simulink model "RocketSimulation"  (R2019b)
settings: Solver=VariableStepAuto  StartTime=0.0  StopTime=10.0  RelTol=1e-3
InitFcn:
  | SimInit;
values from neighbouring files (symbols this model uses):
  AtmoData = [128.186136479 128.244270677 128.302404875 128.485675494 128.734477787 129.006749738 129.455630863 129.904511988 130.470611984 131.122189026 131.781835085 132.638750532 ... (4000 elements, 1000x4)]    [EarthAtmoData.mat]
undefined symbols (not defined in the file or in its folder): Aero_On, AtmoAlt_planet, Cd, Cl, Constant_Drag_On, Constant_Lift_On, Drag_On, DragData, g0, GM_planet, Lift_On, Omega_planet, PitchOverAlt, PitchOverAngle, PitchSwitch, R_planet, RefSurfArea, SimData
libraries: simulink_extras x6, dspmathops x4, vrlib x2, simulink x1
settings Model: Creator=raulm_000  LastModifiedBy=raulm_000

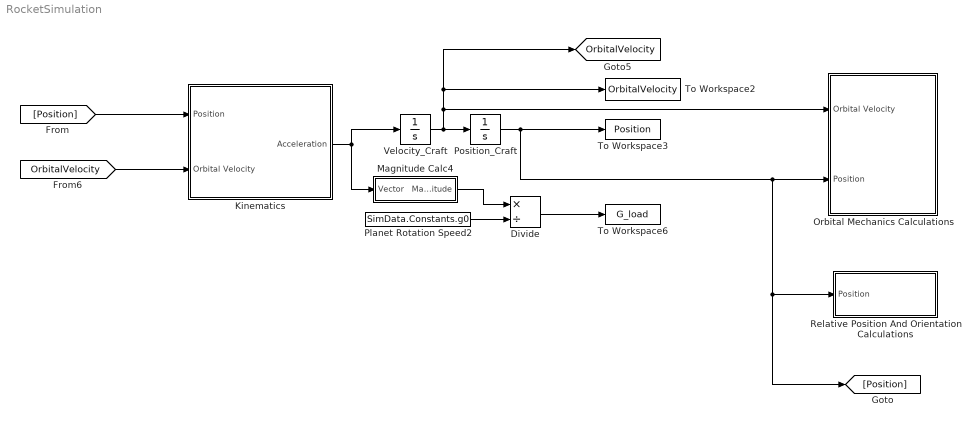
== system RocketSimulation ==
  Divide : Product  Inputs=*/
  Kinematics : Subsystem
  Magnitude Calc4 : Subsystem
  Orbital Mechanics Calculations : Subsystem
  Planet Rotation Speed2 : Constant  Value=SimData.Constants.g0
  Position_Craft : Integrator  InitialCondition=SimData.InitialCondition.P
  Relative Position And Orientation Calculations : Subsystem
  To Workspace2 : ToWorkspace  VariableName=OrbitalVelocity  SampleTime=-1
  To Workspace3 : ToWorkspace  VariableName=Position  SampleTime=-1
  To Workspace6 : ToWorkspace  VariableName=G_load  SampleTime=-1
  Velocity_Craft : Integrator  InitialCondition=SimData.InitialCondition.V
  tag scope: OrbitalVelocity=global
  wires:
  [OrbitalVelocity] -> Kinematics/2(Orbital Velocity)
  Kinematics/1("Acceleration ") -> Velocity_Craft/1, Magnitude Calc4/1(Vector)
  Magnitude Calc4/1("Magnitude ") -> Divide/1
  Planet Rotation Speed2/1 -> Divide/2
  Divide/1 -> To Workspace6/1
  Velocity_Craft/1 -> Position_Craft/1, [OrbitalVelocity], To Workspace2/1, Orbital Mechanics Calculations/1(Orbital Velocity)
  [Position] -> Kinematics/1(Position)
  Position_Craft/1 -> [Position], Relative Position And Orientation Calculations/1(Position), Orbital Mechanics Calculations/2(Position), To Workspace3/1

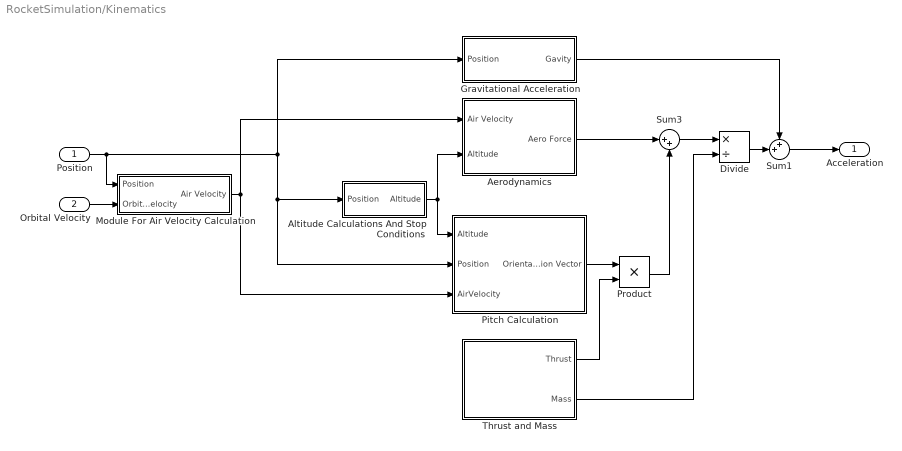
== system RocketSimulation/Kinematics ==
  Position : Inport
  Orbital Velocity : Inport  Port=2
  Aerodynamics : Subsystem
  Altitude Calculations And Stop Conditions : Subsystem
  Divide : Product  Inputs=*/
  Gravitational Acceleration : Subsystem
  Module For Air Velocity Calculation : Subsystem
  Pitch Calculation : Subsystem
  Product : Product
  Sum1 : Sum  Inputs=++|
  Sum3 : Sum  Inputs=|++
  Thrust and Mass : Subsystem
  "Acceleration " : Outport
  wires:
  Position/1 -> Module For Air Velocity Calculation/1(Position), Gravitational Acceleration/1(Position), Pitch Calculation/2(Position), Altitude Calculations And Stop Conditions/1(Position)
  Module For Air Velocity Calculation/1(Air Velocity) -> Pitch Calculation/3(AirVelocity), Aerodynamics/1(Air Velocity)
  Thrust and Mass/1("Thrust ") -> Product/2
  Altitude Calculations And Stop Conditions/1(Altitude) -> Pitch Calculation/1(Altitude), Aerodynamics/2("Altitude ")
  Orbital Velocity/1 -> Module For Air Velocity Calculation/2(Orbital Velocity)
  Pitch Calculation/1(Orientation Vector) -> Product/1
  Aerodynamics/1("Aero Force ") -> Sum3/1
  Product/1 -> Sum3/2
  Sum3/1 -> Divide/1
  Thrust and Mass/2(Mass) -> Divide/2
  Divide/1 -> Sum1/2
  Sum1/1 -> "Acceleration "/1
  Gravitational Acceleration/1("Gavity ") -> Sum1/1

== system RocketSimulation/Magnitude Calc4 ==
  Vector : Inport
  Add : Sum
  Demux : Demux  Outputs=2
  Math Function : Math  Operator=square  SaturateOnIntegerOverflow=on
  Math Function1 : Math  Operator=square  SaturateOnIntegerOverflow=on
  Sqrt : Sqrt  SaturateOnIntegerOverflow=on
  "Magnitude " : Outport
  wires:
  Demux/1 -> Math Function1/1
  Demux/2 -> Math Function/1
  Math Function/1 -> Add/2
  Add/1 -> Sqrt/1
  Vector/1 -> Demux/1
  Math Function1/1 -> Add/1
  Sqrt/1 -> "Magnitude "/1

== system RocketSimulation/Orbital Mechanics Calculations ==
  Orbital Velocity : Inport
  Position : Inport  Port=2
  Gain1 : Gain  Gain=1.01
  MATLAB Function : MATLAB Function  TreatAsAtomicUnit=on
  Planet Rotation Speed4 : Constant  Value=SimData.TargetOrbit
  Relational Operator : RelationalOperator  OutDataTypeStr=boolean  RndMeth=Nearest
  tag scope: TOR=global
  wires:
  Planet Rotation Speed4/1 -> Gain1/1
  Relational Operator/1 -> [TOR]
  Gain1/1 -> Relational Operator/2
  Orbital Velocity/1 -> MATLAB Function/1(OrbitVelocity)
  Position/1 -> MATLAB Function/2(Position)

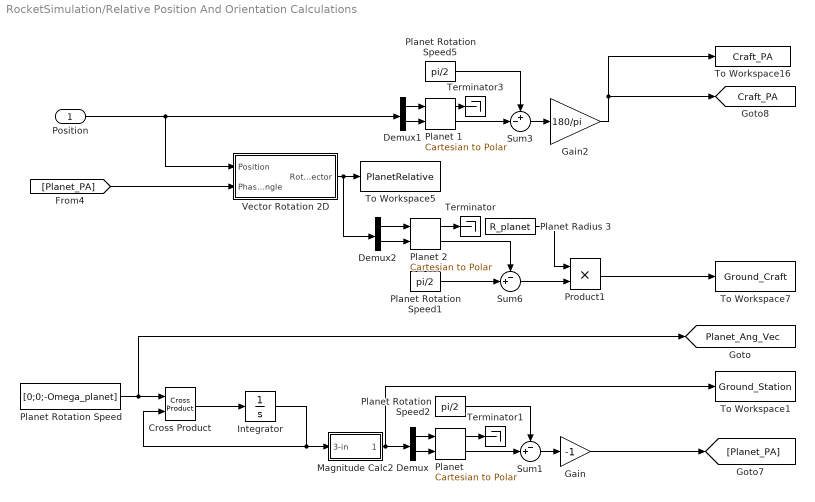
== system RocketSimulation/Relative Position And Orientation Calculations ==
  Position : Inport
  Cross Product : vrlib/Utilities/Cross Product
      settings: SourceProductName=Simulink
  Demux : Demux  Outputs=2
  Demux1 : Demux  Outputs=2
  Demux2 : Demux  Outputs=2
  Gain : Gain  Gain=-1
  Gain2 : Gain  Gain=180/pi
  Integrator : Integrator  InitialCondition=[0;R_planet;0]
  Magnitude Calc2 : Subsystem
  "Planet " : simulink_extras/Transformations/Cartesian to Polar
      settings: SourceProductName=Simulink
  Planet 1 : simulink_extras/Transformations/Cartesian to Polar
      settings: SourceProductName=Simulink
  Planet 2 : simulink_extras/Transformations/Cartesian to Polar
      settings: SourceProductName=Simulink
  Planet Radius 3 : Constant  Value=R_planet
  Planet Rotation Speed : Constant  Value=[0;0;-Omega_planet]
  Planet Rotation Speed1 : Constant  Value=pi/2
  Planet Rotation Speed2 : Constant  Value=pi/2
  Planet Rotation Speed5 : Constant  Value=pi/2
  Product1 : Product
  Sum1 : Sum  Inputs=-+|
  Sum3 : Sum  Inputs=+-|
  Sum6 : Sum  Inputs=-+|
  Terminator : Terminator
  Terminator1 : Terminator
  Terminator3 : Terminator
  To Workspace1 : ToWorkspace  VariableName=Ground_Station  SampleTime=-1
  To Workspace16 : ToWorkspace  VariableName=Craft_PA  SampleTime=-1
  To Workspace5 : ToWorkspace  VariableName=PlanetRelative  SampleTime=-1
  To Workspace7 : ToWorkspace  VariableName=Ground_Craft  SampleTime=-1
  Vector Rotation 2D : Subsystem
  tag scope: Craft_PA=global, Planet_Ang_Vec=global
  wires:
  Planet Rotation Speed/1 -> [Planet_Ang_Vec], Cross Product/1
  Integrator/1 -> Cross Product/2, Magnitude Calc2/1(3-in)
  Cross Product/1 -> Integrator/1
  Magnitude Calc2/1("2-out ") -> To Workspace1/1, Demux/1
  Demux/1 -> "Planet "/1
  Demux/2 -> "Planet "/2
  Vector Rotation 2D/1("Rotated Vector ") -> Demux2/1, To Workspace5/1
  "Planet "/2 -> Sum1/2
  Planet Rotation Speed2/1 -> Sum1/1
  Sum1/1 -> Gain/1
  Planet 2/2 -> Sum6/1
  Planet Radius 3/1 -> Product1/1
  Product1/1 -> To Workspace7/1
  Planet Rotation Speed1/1 -> Sum6/2
  Sum6/1 -> Product1/2
  Demux2/1 -> Planet 2/1
  Demux2/2 -> Planet 2/2
  Planet 2/1 -> Terminator/1
  "Planet "/1 -> Terminator1/1
  Gain/1 -> [Planet_PA]
  [Planet_PA] -> Vector Rotation 2D/2(Phase Angle)
  Demux1/1 -> Planet 1/1
  Demux1/2 -> Planet 1/2
  Planet 1/2 -> Sum3/2
  Planet Rotation Speed5/1 -> Sum3/1
  Planet 1/1 -> Terminator3/1
  Sum3/1 -> Gain2/1
  Gain2/1 -> To Workspace16/1, [Craft_PA]
  Position/1 -> Vector Rotation 2D/1(Position), Demux1/1

== system RocketSimulation/Kinematics/Aerodynamics ==
  Air Velocity : Inport
  "Altitude " : Inport  Port=2
  Add : Sum  Inputs=+-
  Aerodynamic Calculations : Subsystem
  Atmosphere Max Alt : Constant  Value=AtmoAlt_planet
  Constant1 : Constant  Value=0
  Constant2 : Constant  Value=Aero_On
  Constant3 : Constant  Value=0
  Switch : Switch  Criteria=u2 > Threshold
  Switch1 : Switch  Criteria=u2 ~= 0
  "Aero Force " : Outport
  wires:
  "Altitude "/1 -> Aerodynamic Calculations/2(Altitude), Add/2
  Atmosphere Max Alt/1 -> Add/1
  Add/1 -> Switch/2
  Constant1/1 -> Switch/3
  Switch1/1 -> "Aero Force "/1
  Air Velocity/1 -> Aerodynamic Calculations/1(Air Velocity)
  Aerodynamic Calculations/1("Aeroforce ") -> Switch/1
  Switch/1 -> Switch1/3
  Constant2/1 -> Switch1/2
  Constant3/1 -> Switch1/1

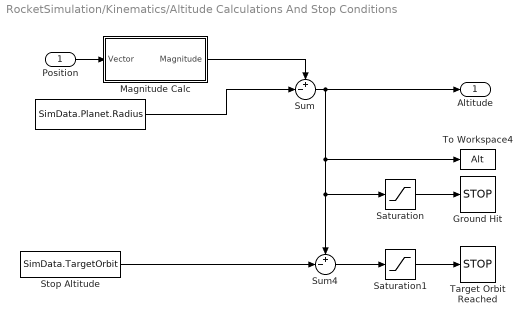
== system RocketSimulation/Kinematics/Altitude Calculations And Stop Conditions ==
  Position : Inport
  " " : Constant  Value=SimData.Planet.Radius
  " Target Orbit Reached" : Stop
  Ground Hit : Stop
  Magnitude Calc : Subsystem
  Saturation : Saturate  UpperLimit=0
  Saturation1 : Saturate  UpperLimit=1  LowerLimit=0
  Stop Altitude : Constant  Value=SimData.TargetOrbit
  Sum : Sum  Inputs=+-|
  Sum4 : Sum  Inputs=+-|
  To Workspace4 : ToWorkspace  VariableName=Alt  SampleTime=-1
  Altitude : Outport
  wires:
  Magnitude Calc/1("Magnitude ") -> Sum/1
  " "/1 -> Sum/2
  Sum/1 -> Sum4/1, Saturation/1, To Workspace4/1, Altitude/1
  Saturation/1 -> Ground Hit/1
  Stop Altitude/1 -> Sum4/2
  Sum4/1 -> Saturation1/1
  Saturation1/1 -> " Target Orbit Reached"/1
  Position/1 -> Magnitude Calc/1(Vector)

== system RocketSimulation/Kinematics/Gravitational Acceleration ==
  Position : Inport
  Divide : Product  Inputs=*/
  Gain : Gain  Gain=-1
  Magnitude Calc : Subsystem
  Math Function : Math  Operator=square  SaturateOnIntegerOverflow=on
  Normalization : dspmathops/Normalization  NormType=2-norm  Bias=1e-10  NormOver=Specified dimension  Dimension=1  roundingMode=Floor  overflowMode=off  accumDataTypeStr=Inherit: Same as product output  accumLastDataTypeStr=Inherit: Same as product output  outputDataTypeStr=Inherit: Same as product output  outputMin=[]  outputMax=[]  outputLastDataTypeStr=Inherit: Same as product output
      settings: SourceProductName=DSP System Toolbox
  Planet GM : Constant  Value=GM_planet
  Product : Product
  "Gavity " : Outport
  wires:
  Position/1 -> Normalization/1, Magnitude Calc/1(Vector)
  Magnitude Calc/1("Magnitude ") -> Math Function/1
  Planet GM/1 -> Divide/1
  Math Function/1 -> Divide/2
  Product/1 -> "Gavity "/1
  Gain/1 -> Product/2
  Divide/1 -> Product/1
  Normalization/1 -> Gain/1

== system RocketSimulation/Kinematics/Module For Air Velocity Calculation ==
  Position : Inport
  Orbital Velocity : Inport  Port=2
  Cross Product1 : vrlib/Utilities/Cross Product
      settings: SourceProductName=Simulink
  Magnitude Calc3 : Subsystem
  Mux : Mux  Inputs=2
  Planet Rotation Speed1 : Constant  Value=0
  Sum2 : Sum  Inputs=|-+
  Air Velocity : Outport
  wires:
  [Planet_Ang_Vec] -> Cross Product1/1
  Cross Product1/1 -> Magnitude Calc3/1(3-in)
  Mux/1 -> Cross Product1/2
  Planet Rotation Speed1/1 -> Mux/2
  Magnitude Calc3/1("2-out ") -> Sum2/1
  Orbital Velocity/1 -> Sum2/2
  Position/1 -> Mux/1
  Sum2/1 -> Air Velocity/1

== system RocketSimulation/Kinematics/Pitch Calculation ==
  Altitude : Inport  PortDimensions=1
  Position : Inport  Port=2
  AirVelocity : Inport  Port=3
  Constant : Constant  Value=PitchOverAlt
  Gravity Turn Pitch Calculation : Subsystem
  Relational Operator : RelationalOperator  OutDataTypeStr=boolean  RndMeth=Nearest
  Subsystem : Subsystem
  Switch1 : Switch  Criteria=u2 ~= 0  Threshold=PitchOverAlt
  Orientation Vector : Outport
  wires:
  Relational Operator/1 -> Switch1/2
  Constant/1 -> Relational Operator/1
  Altitude/1 -> Subsystem/2(Altitude), Relational Operator/2
  Switch1/1 -> Orientation Vector/1
  Position/1 -> Subsystem/1(Position)
  Subsystem/1(Up Vector) -> Switch1/1
  AirVelocity/1 -> Gravity Turn Pitch Calculation/1(Air Velocity)
  Gravity Turn Pitch Calculation/1(Thrust Vec) -> Switch1/3

== system RocketSimulation/Kinematics/Thrust and Mass ==
  Mass and fuel consumption : Subsystem
  To Workspace1 : ToWorkspace  VariableName=Mass  SampleTime=-1
  "Thrust " : Outport
  Mass : Outport  Port=2
  wires:
  Mass and fuel consumption/1("Thrust ") -> "Thrust "/1
  Mass and fuel consumption/2("Mass ") -> To Workspace1/1, Mass/1

== system RocketSimulation/Relative Position And Orientation Calculations/Magnitude Calc2 ==
  3-in : Inport
  Demux4 : Demux  Outputs=3
  Mux2 : Mux  Inputs=2
  Terminator3 : Terminator
  "2-out " : Outport
  wires:
  3-in/1 -> Demux4/1
  Demux4/3 -> Terminator3/1
  Demux4/1 -> Mux2/1
  Demux4/2 -> Mux2/2
  Mux2/1 -> "2-out "/1

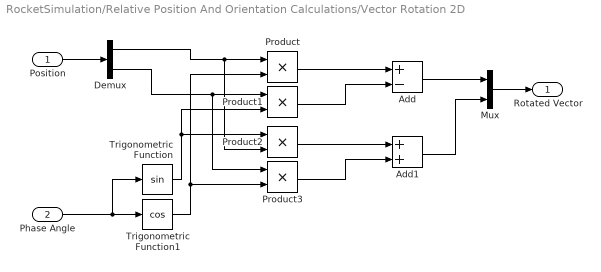
== system RocketSimulation/Relative Position And Orientation Calculations/Vector Rotation 2D ==
  Position : Inport
  Phase Angle : Inport  Port=2
  Add : Sum  Inputs=+-
  Add1 : Sum
  Demux : Demux  Outputs=2
  Mux : Mux  Inputs=2
  Product{,1..3} (4 alike) : Product
  Trigonometric Function : Trigonometry
  Trigonometric Function1 : Trigonometry  Operator=cos
  "Rotated Vector " : Outport
  wires:
  Mux/1 -> "Rotated Vector "/1
  Phase Angle/1 -> Trigonometric Function/1, Trigonometric Function1/1
  Position/1 -> Demux/1
  Trigonometric Function1/1 -> Product3/2, Product/2
  Demux/1 -> Product2/2, Product/1
  Product/1 -> Add/1
  Demux/2 -> Product3/1, Product1/1
  Trigonometric Function/1 -> Product2/1, Product1/2
  Product1/1 -> Add/2
  Product2/1 -> Add1/1
  Product3/1 -> Add1/2
  Add1/1 -> Mux/2
  Add/1 -> Mux/1

== system RocketSimulation/Kinematics/Aerodynamics/Aerodynamic Calculations ==
  Air Velocity : Inport
  Altitude : Inport  Port=2
  Cl and Cd Calculation : Subsystem
  Magnitude Calc1 : Subsystem
  Product : Product  Inputs=3
  Referance Surface Area : Constant  Value=RefSurfArea
  "Aeroforce " : Outport
  wires:
  Air Velocity/1 -> Cl and Cd Calculation/1(Air Velocity), Magnitude Calc1/1(Air Velocity)
  Altitude/1 -> Cl and Cd Calculation/2("Altitude "), Magnitude Calc1/2("Altitude ")
  Product/1 -> "Aeroforce "/1
  Magnitude Calc1/1("Dynamic Pressure ") -> Product/1
  Cl and Cd Calculation/1(Cl + Cd) -> Product/2
  Referance Surface Area/1 -> Product/3

== system RocketSimulation/Kinematics/Altitude Calculations And Stop Conditions/Magnitude Calc ==
  Vector : Inport
  Add : Sum
  Demux : Demux  Outputs=2
  Math Function : Math  Operator=square  SaturateOnIntegerOverflow=on
  Math Function1 : Math  Operator=square  SaturateOnIntegerOverflow=on
  Sqrt : Sqrt  SaturateOnIntegerOverflow=on
  "Magnitude " : Outport
  wires:
  Demux/1 -> Math Function1/1
  Demux/2 -> Math Function/1
  Math Function/1 -> Add/2
  Add/1 -> Sqrt/1
  Vector/1 -> Demux/1
  Math Function1/1 -> Add/1
  Sqrt/1 -> "Magnitude "/1

== system RocketSimulation/Kinematics/Gravitational Acceleration/Magnitude Calc ==
  Vector : Inport
  Add : Sum
  Demux : Demux  Outputs=2
  Math Function : Math  Operator=square  SaturateOnIntegerOverflow=on
  Math Function1 : Math  Operator=square  SaturateOnIntegerOverflow=on
  Sqrt : Sqrt  SaturateOnIntegerOverflow=on
  "Magnitude " : Outport
  wires:
  Demux/1 -> Math Function1/1
  Demux/2 -> Math Function/1
  Math Function/1 -> Add/2
  Add/1 -> Sqrt/1
  Vector/1 -> Demux/1
  Math Function1/1 -> Add/1
  Sqrt/1 -> "Magnitude "/1

== system RocketSimulation/Kinematics/Module For Air Velocity Calculation/Magnitude Calc3 ==
  3-in : Inport
  Demux4 : Demux  Outputs=3
  Mux2 : Mux  Inputs=2
  Terminator3 : Terminator
  "2-out " : Outport
  wires:
  3-in/1 -> Demux4/1
  Demux4/3 -> Terminator3/1
  Demux4/1 -> Mux2/1
  Demux4/2 -> Mux2/2
  Mux2/1 -> "2-out "/1

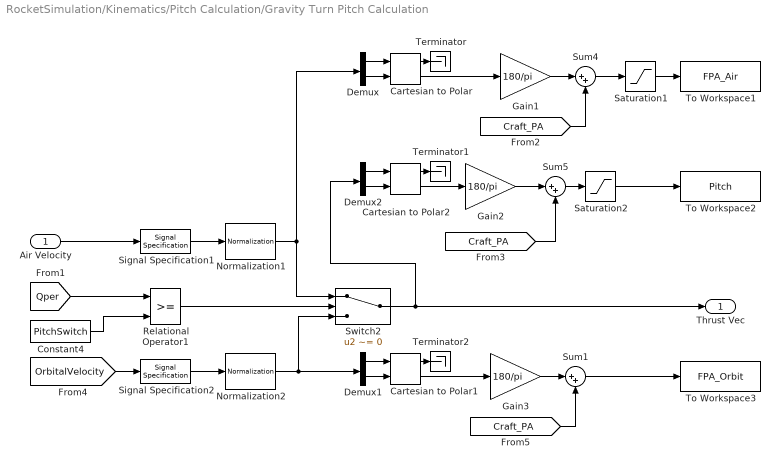
== system RocketSimulation/Kinematics/Pitch Calculation/Gravity Turn Pitch Calculation ==
  Air Velocity : Inport
  Cartesian to Polar : simulink_extras/Transformations/Cartesian to Polar
      settings: SourceProductName=Simulink
  Cartesian to Polar1 : simulink_extras/Transformations/Cartesian to Polar
      settings: SourceProductName=Simulink
  Cartesian to Polar2 : simulink_extras/Transformations/Cartesian to Polar
      settings: SourceProductName=Simulink
  Constant4 : Constant  Value=PitchSwitch
  Demux : Demux  Outputs=2
  Demux1 : Demux  Outputs=2
  Demux2 : Demux  Outputs=2
  Gain1 : Gain  Gain=180/pi
  Gain2 : Gain  Gain=180/pi
  Gain3 : Gain  Gain=180/pi
  Normalization1 : dspmathops/Normalization  NormType=2-norm  Bias=1e-10  NormOver=Specified dimension  Dimension=1  roundingMode=Floor  overflowMode=off  accumDataTypeStr=Inherit: Same as product output  accumLastDataTypeStr=Inherit: Same as product output  outputMin=[]  outputMax=[]
      settings: SourceProductName=DSP System Toolbox
  Normalization2 : dspmathops/Normalization  NormType=2-norm  Bias=1e-10  NormOver=Specified dimension  Dimension=1  roundingMode=Floor  overflowMode=off  accumDataTypeStr=Inherit: Same as product output  accumLastDataTypeStr=Inherit: Same as product output  outputMin=[]  outputMax=[]
      settings: SourceProductName=DSP System Toolbox
  Relational Operator1 : RelationalOperator  OutDataTypeStr=boolean  RndMeth=Nearest
  Saturation1 : Saturate  UpperLimit=90  LowerLimit=0
  Saturation2 : Saturate  UpperLimit=90  LowerLimit=0
  Signal Specification1 : SignalSpecification  Dimensions=2
  Signal Specification2 : SignalSpecification  Dimensions=2
  Sum1 : Sum  Inputs=|++
  Sum4 : Sum  Inputs=|++
  Sum5 : Sum  Inputs=|++
  Switch2 : Switch  Criteria=u2 ~= 0  Threshold=PitchOverAlt
  Terminator : Terminator
  Terminator1 : Terminator
  Terminator2 : Terminator
  To Workspace1 : ToWorkspace  VariableName=FPA_Air  SampleTime=-1
  To Workspace2 : ToWorkspace  VariableName=Pitch  SampleTime=-1
  To Workspace3 : ToWorkspace  VariableName=FPA_Orbit  SampleTime=-1
  Thrust Vec : Outport
  wires:
  [Qper] -> Relational Operator1/1
  Relational Operator1/1 -> Switch2/2
  Normalization1/1 -> Switch2/1, Demux/1
  Demux1/1 -> Cartesian to Polar1/1
  Switch2/1 -> Thrust Vec/1, Demux2/1
  Constant4/1 -> Relational Operator1/2
  Cartesian to Polar/1 -> Terminator/1
  Sum1/1 -> To Workspace3/1
  Air Velocity/1 -> Signal Specification1/1
  Demux/2 -> Cartesian to Polar/2
  Signal Specification2/1 -> Normalization2/1
  Normalization2/1 -> Demux1/1, Switch2/3
  Signal Specification1/1 -> Normalization1/1
  Demux/1 -> Cartesian to Polar/1
  Demux1/2 -> Cartesian to Polar1/2
  Cartesian to Polar1/1 -> Terminator2/1
  [OrbitalVelocity] -> Signal Specification2/1
  Gain1/1 -> Sum4/1
  Cartesian to Polar1/2 -> Gain3/1
  Gain3/1 -> Sum1/1
  [Craft_PA] -> Sum1/2
  Saturation2/1 -> To Workspace2/1
  Cartesian to Polar/2 -> Gain1/1
  Cartesian to Polar2/1 -> Terminator1/1
  Saturation1/1 -> To Workspace1/1
  Gain2/1 -> Sum5/1
  [Craft_PA] -> Sum5/2
  Sum5/1 -> Saturation2/1
  Demux2/1 -> Cartesian to Polar2/1
  Cartesian to Polar2/2 -> Gain2/1
  Demux2/2 -> Cartesian to Polar2/2
  [Craft_PA] -> Sum4/2
  Sum4/1 -> Saturation1/1

== system RocketSimulation/Kinematics/Pitch Calculation/Subsystem ==
  Position : Inport
  Altitude : Inport  Port=2
  Gain : Gain  Gain=-pi/180
  Linear Pitch Over : Gain  Gain=PitchOverAngle/PitchOverAlt
  Normalization : dspmathops/Normalization  NormType=2-norm  Bias=1e-10  NormOver=Specified dimension  Dimension=1  roundingMode=Floor  overflowMode=off  accumDataTypeStr=Inherit: Same as product output  accumLastDataTypeStr=Inherit: Same as product output  outputMin=[]  outputMax=[]
      settings: SourceProductName=DSP System Toolbox
  Saturation : Saturate  UpperLimit=90  LowerLimit=0
  Signal Specification : SignalSpecification  Dimensions=2
  Vector Rotation 2D : Subsystem
  Up Vector : Outport
  wires:
  Altitude/1 -> Linear Pitch Over/1
  Position/1 -> Signal Specification/1
  Signal Specification/1 -> Normalization/1
  Normalization/1 -> Vector Rotation 2D/1(Position)
  Saturation/1 -> Gain/1
  Gain/1 -> Vector Rotation 2D/2(Phase Angle)
  Linear Pitch Over/1 -> Saturation/1
  Vector Rotation 2D/1("Rotated Vector ") -> Up Vector/1

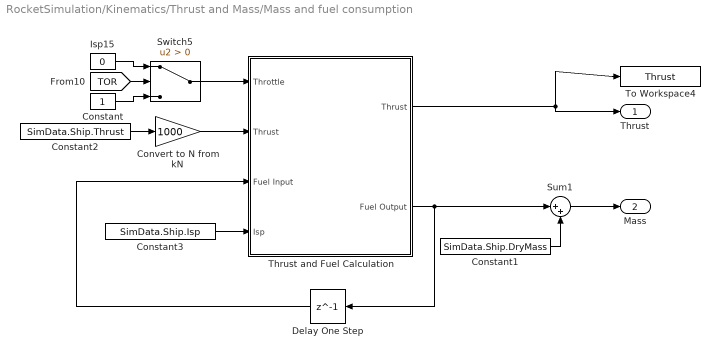
== system RocketSimulation/Kinematics/Thrust and Mass/Mass and fuel consumption ==
  Constant : Constant
  Constant1 : Constant  Value=SimData.Ship.DryMass
  Constant2 : Constant  Value=SimData.Ship.Thrust
  Constant3 : Constant  Value=SimData.Ship.Isp
  Convert to N from kN : Gain  Gain=1000
  Delay One Step : Delay  DelayLength=1
  Isp15 : Constant  Value=0
  Sum1 : Sum  Inputs=|++
  Switch5 : Switch  Criteria=u2 > Threshold
  Thrust and Fuel Calculation : Subsystem
  To Workspace4 : ToWorkspace  VariableName=Thrust  SampleTime=-1
      settings: MaxDataPoints=1
  "Thrust " : Outport
  "Mass " : Outport  Port=2
  wires:
  Sum1/1 -> "Mass "/1
  Convert to N from kN/1 -> Thrust and Fuel Calculation/2(Thrust)
  Thrust and Fuel Calculation/1("Thrust ") -> "Thrust "/1, To Workspace4/1
  Thrust and Fuel Calculation/2(Fuel Output) -> Delay One Step/1, Sum1/1
  Isp15/1 -> Switch5/1
  [TOR] -> Switch5/2
  Constant/1 -> Switch5/3
  Switch5/1 -> Thrust and Fuel Calculation/1(Throttle)
  Delay One Step/1 -> Thrust and Fuel Calculation/3(Fuel Input)
  Constant1/1 -> Sum1/2
  Constant2/1 -> Convert to N from kN/1
  Constant3/1 -> Thrust and Fuel Calculation/4(Isp)

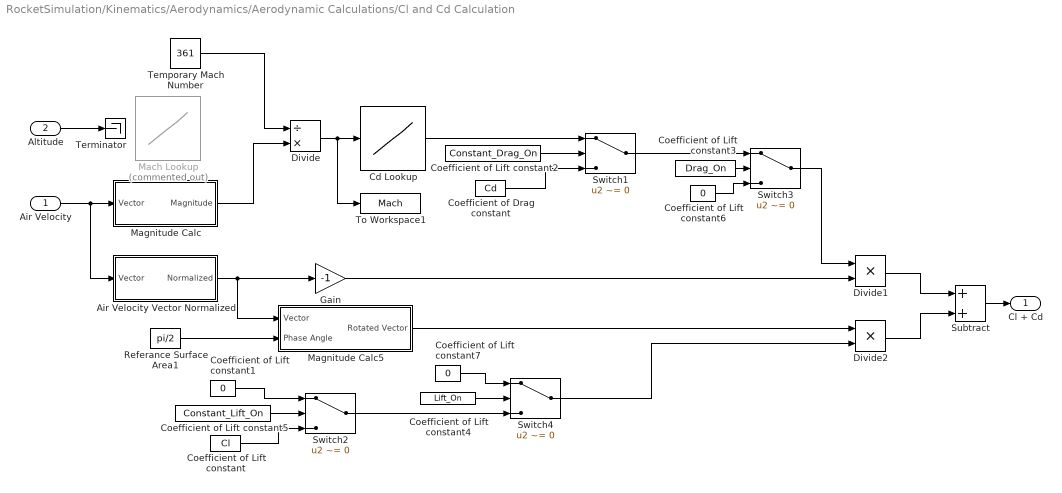
== system RocketSimulation/Kinematics/Aerodynamics/Aerodynamic Calculations/Cl and Cd Calculation ==
  Air Velocity : Inport
  "Altitude " : Inport  Port=2
  Air Velocity Vector Normalized : Subsystem
  Cd Lookup : Lookup_n-D  NumberOfTableDimensions=1  BreakpointsForDimension1=DragData(:,1)  Table=DragData(:,2)  InternalRulePriority=Speed  RndMeth=Simplest  InputSameDT=on
  Coefficient of Drag constant : Constant  Value=Cd
  Coefficient of Lift constant : Constant  Value=Cl
  Coefficient of Lift constant1 : Constant  Value=0
  Coefficient of Lift constant2 : Constant  Value=Constant_Drag_On
  Coefficient of Lift constant3 : Constant  Value=Drag_On
  Coefficient of Lift constant4 : Constant  Value=Lift_On
  Coefficient of Lift constant5 : Constant  Value=Constant_Lift_On
  Coefficient of Lift constant6 : Constant  Value=0
  Coefficient of Lift constant7 : Constant  Value=0
  Divide : Product  Inputs=/*
  Divide1 : Product  Inputs=**
  Divide2 : Product  Inputs=**
  Gain : Gain  Gain=-1
  Mach Lookup : Lookup_n-D  Commented=on  NumberOfTableDimensions=1  BreakpointsForDimension1=AtmoData(:,1)  Table=AtmoData(:,4)  InternalRulePriority=Speed  RndMeth=Simplest  InputSameDT=on
  Magnitude Calc : Subsystem
  Magnitude Calc5 : Subsystem
  Referance Surface Area1 : Constant  Value=pi/2
  Subtract : Sum
  Switch{1..4} (4 alike) : Switch  Criteria=u2 ~= 0
  Temporary Mach Number : Constant  Value=361
  Terminator : Terminator
  To Workspace1 : ToWorkspace  VariableName=Mach  SampleTime=-1
  Cl + Cd : Outport
  wires:
  Air Velocity/1 -> Air Velocity Vector Normalized/1(Vector), Magnitude Calc/1(Vector)
  Magnitude Calc/1("Magnitude ") -> Divide/2
  Divide/1 -> To Workspace1/1, Cd Lookup/1
  Air Velocity Vector Normalized/1("Normalized ") -> Magnitude Calc5/1(Vector), Gain/1
  Gain/1 -> Divide1/2
  Divide1/1 -> Subtract/1
  Referance Surface Area1/1 -> Magnitude Calc5/2(Phase Angle)
  Magnitude Calc5/1("Rotated Vector ") -> Divide2/1
  Coefficient of Lift constant2/1 -> Switch1/2
  Switch3/1 -> Divide1/1
  Subtract/1 -> Cl + Cd/1
  Coefficient of Drag constant/1 -> Switch1/3
  Cd Lookup/1 -> Switch1/1
  Coefficient of Lift constant5/1 -> Switch2/2
  Coefficient of Lift constant1/1 -> Switch2/1
  Coefficient of Lift constant/1 -> Switch2/3
  Coefficient of Lift constant3/1 -> Switch3/2
  Coefficient of Lift constant6/1 -> Switch3/3
  Switch1/1 -> Switch3/1
  Coefficient of Lift constant4/1 -> Switch4/2
  Switch2/1 -> Switch4/3
  Coefficient of Lift constant7/1 -> Switch4/1
  Switch4/1 -> Divide2/2
  Divide2/1 -> Subtract/2
  "Altitude "/1 -> Terminator/1
  Temporary Mach Number/1 -> Divide/1

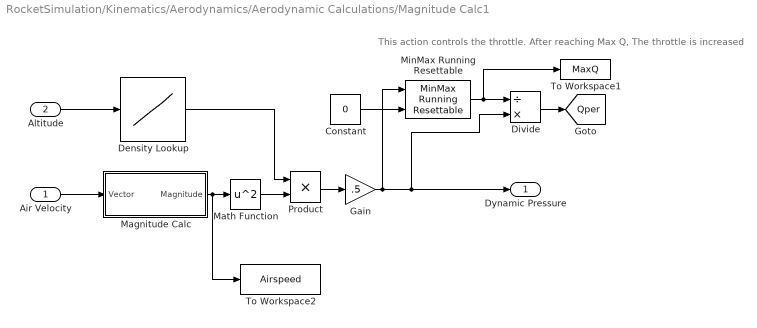
== system RocketSimulation/Kinematics/Aerodynamics/Aerodynamic Calculations/Magnitude Calc1 ==
  note: This action controls the throttle. After reaching Max Q, The throttle is increased
  Air Velocity : Inport
  "Altitude " : Inport  Port=2
  Constant : Constant  Value=0
  Density Lookup : Lookup_n-D  NumberOfTableDimensions=1  BreakpointsForDimension1=AtmoData(:,1)  Table=AtmoData(:,3)  InternalRulePriority=Speed  RndMeth=Simplest  InputSameDT=on
  Divide : Product  Inputs=/*
  Gain : Gain  Gain=.5
  Magnitude Calc : Subsystem
  Math Function : Math  Operator=square  SaturateOnIntegerOverflow=on
  MinMax Running Resettable : simulink/Math Operations/MinMax Running Resettable  Function=max  vinit=0.0
  Product : Product
  To Workspace1 : ToWorkspace  VariableName=MaxQ  SampleTime=-1
      settings: MaxDataPoints=1
  To Workspace2 : ToWorkspace  VariableName=Airspeed  SampleTime=-1
  "Dynamic Pressure " : Outport
  tag scope: Qper=global
  wires:
  "Altitude "/1 -> Density Lookup/1
  Magnitude Calc/1("Magnitude ") -> To Workspace2/1, Math Function/1
  Air Velocity/1 -> Magnitude Calc/1(Vector)
  Math Function/1 -> Product/2
  Product/1 -> Gain/1
  Density Lookup/1 -> Product/1
  MinMax Running Resettable/1 -> To Workspace1/1, Divide/1
  Constant/1 -> MinMax Running Resettable/2
  Gain/1 -> MinMax Running Resettable/1, Divide/2, "Dynamic Pressure "/1
  Divide/1 -> [Qper]

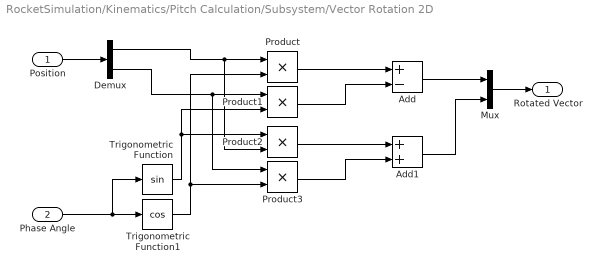
== system RocketSimulation/Kinematics/Pitch Calculation/Subsystem/Vector Rotation 2D ==
  Position : Inport
  Phase Angle : Inport  Port=2
  Add : Sum  Inputs=+-
  Add1 : Sum
  Demux : Demux  Outputs=2
  Mux : Mux  Inputs=2
  Product{,1..3} (4 alike) : Product
  Trigonometric Function : Trigonometry
  Trigonometric Function1 : Trigonometry  Operator=cos
  "Rotated Vector " : Outport
  wires:
  Mux/1 -> "Rotated Vector "/1
  Phase Angle/1 -> Trigonometric Function/1, Trigonometric Function1/1
  Position/1 -> Demux/1
  Trigonometric Function1/1 -> Product3/2, Product/2
  Demux/1 -> Product2/2, Product/1
  Product/1 -> Add/1
  Demux/2 -> Product3/1, Product1/1
  Trigonometric Function/1 -> Product2/1, Product1/2
  Product1/1 -> Add/2
  Product2/1 -> Add1/1
  Product3/1 -> Add1/2
  Add1/1 -> Mux/2
  Add/1 -> Mux/1

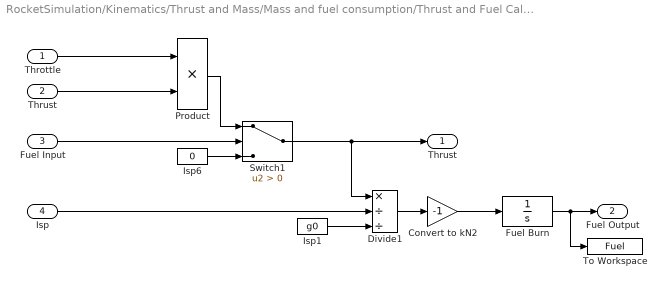
== system RocketSimulation/Kinematics/Thrust and Mass/Mass and fuel consumption/Thrust and Fuel Calculation ==
  Throttle : Inport
  Thrust : Inport  Port=2
  Fuel Input : Inport  Port=3
  Isp : Inport  Port=4
  Convert to kN2 : Gain  Gain=-1
  Divide1 : Product  Inputs=*//
  Fuel Burn : Integrator  InitialCondition=SimData.Ship.WetMass - SimData.Ship.DryMass  LimitOutput=on  LowerSaturationLimit=0
  Isp1 : Constant  Value=g0
  Isp6 : Constant  Value=0
  Product : Product
  Switch1 : Switch  Criteria=u2 > Threshold
  To Workspace : ToWorkspace  VariableName=Fuel  SampleTime=-1
      settings: MaxDataPoints=1
  "Thrust " : Outport
  Fuel Output : Outport  Port=2
  wires:
  Isp1/1 -> Divide1/3
  Divide1/1 -> Convert to kN2/1
  Convert to kN2/1 -> Fuel Burn/1
  Thrust/1 -> Product/2
  Product/1 -> Switch1/1
  Throttle/1 -> Product/1
  Switch1/1 -> Divide1/1, "Thrust "/1
  Isp6/1 -> Switch1/3
  Isp/1 -> Divide1/2
  Fuel Input/1 -> Switch1/2
  Fuel Burn/1 -> Fuel Output/1, To Workspace/1

== system RocketSimulation/Kinematics/Aerodynamics/Aerodynamic Calculations/Cl and Cd Calculation/Air Velocity Vector Normalized ==
  Vector : Inport
  Constant : Constant
  Demux3 : Demux  Outputs=2
  Divide1 : Product  Inputs=*/
  Divide2 : Product  Inputs=*/
  Magnitude Calc : Subsystem
  Mux1 : Mux  Inputs=2
  Switch : Switch  Criteria=u2 > Threshold
  "Normalized " : Outport
  wires:
  Demux3/1 -> Divide1/1
  Vector/1 -> Demux3/1, Magnitude Calc/1(Vector)
  Mux1/1 -> "Normalized "/1
  Demux3/2 -> Divide2/1
  Constant/1 -> Switch/3
  Magnitude Calc/1("Magnitude ") -> Switch/1
  Magnitude Calc/2(Is Zero) -> Switch/2
  Divide1/1 -> Mux1/1
  Divide2/1 -> Mux1/2
  Switch/1 -> Divide2/2, Divide1/2

== system RocketSimulation/Kinematics/Aerodynamics/Aerodynamic Calculations/Cl and Cd Calculation/Magnitude Calc ==
  Vector : Inport
  Add : Sum
  Demux : Demux  Outputs=2
  Math Function : Math  Operator=square  SaturateOnIntegerOverflow=on
  Math Function1 : Math  Operator=square  SaturateOnIntegerOverflow=on
  Sqrt : Sqrt  SaturateOnIntegerOverflow=on
  "Magnitude " : Outport
  wires:
  Demux/1 -> Math Function1/1
  Demux/2 -> Math Function/1
  Math Function/1 -> Add/2
  Add/1 -> Sqrt/1
  Vector/1 -> Demux/1
  Math Function1/1 -> Add/1
  Sqrt/1 -> "Magnitude "/1

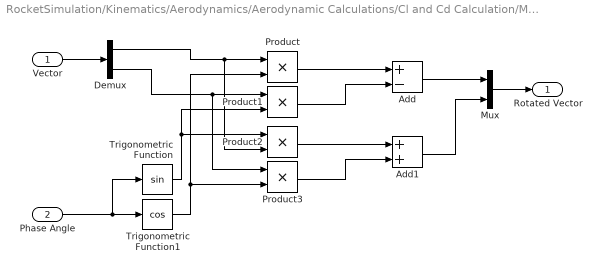
== system RocketSimulation/Kinematics/Aerodynamics/Aerodynamic Calculations/Cl and Cd Calculation/Magnitude Calc5 ==
  Vector : Inport
  Phase Angle : Inport  Port=2
  Add : Sum  Inputs=+-
  Add1 : Sum
  Demux : Demux  Outputs=2
  Mux : Mux  Inputs=2
  Product{,1..3} (4 alike) : Product
  Trigonometric Function : Trigonometry
  Trigonometric Function1 : Trigonometry  Operator=cos
  "Rotated Vector " : Outport
  wires:
  Mux/1 -> "Rotated Vector "/1
  Phase Angle/1 -> Trigonometric Function/1, Trigonometric Function1/1
  Vector/1 -> Demux/1
  Trigonometric Function1/1 -> Product3/2, Product/2
  Demux/1 -> Product2/2, Product/1
  Product/1 -> Add/1
  Demux/2 -> Product3/1, Product1/1
  Trigonometric Function/1 -> Product2/1, Product1/2
  Product1/1 -> Add/2
  Product2/1 -> Add1/1
  Product3/1 -> Add1/2
  Add1/1 -> Mux/2
  Add/1 -> Mux/1

== system RocketSimulation/Kinematics/Aerodynamics/Aerodynamic Calculations/Magnitude Calc1/Magnitude Calc ==
  Vector : Inport
  Add : Sum
  Demux : Demux  Outputs=2
  Math Function : Math  Operator=square  SaturateOnIntegerOverflow=on
  Math Function1 : Math  Operator=square  SaturateOnIntegerOverflow=on
  Sqrt : Sqrt  SaturateOnIntegerOverflow=on
  "Magnitude " : Outport
  wires:
  Demux/1 -> Math Function1/1
  Demux/2 -> Math Function/1
  Math Function/1 -> Add/2
  Add/1 -> Sqrt/1
  Vector/1 -> Demux/1
  Math Function1/1 -> Add/1
  Sqrt/1 -> "Magnitude "/1

== system RocketSimulation/Kinematics/Aerodynamics/Aerodynamic Calculations/Cl and Cd Calculation/Air Velocity Vector Normalized/Magnitude Calc ==
  Vector : Inport
  Add : Sum
  Constant : Constant
  Constant1 : Constant  Value=0
  Demux : Demux  Outputs=2
  Math Function : Math  Operator=square  SaturateOnIntegerOverflow=on
  Math Function1 : Math  Operator=square  SaturateOnIntegerOverflow=on
  Sqrt : Sqrt  SaturateOnIntegerOverflow=on
  Switch : Switch  Criteria=u2 ~= 0
  "Magnitude " : Outport
  Is Zero : Outport  Port=2
  wires:
  Demux/1 -> Math Function1/1
  Demux/2 -> Math Function/1
  Math Function/1 -> Add/2
  Add/1 -> Sqrt/1
  Vector/1 -> Demux/1
  Math Function1/1 -> Add/1
  Switch/1 -> Is Zero/1
  Constant/1 -> Switch/1
  Constant1/1 -> Switch/3
  Sqrt/1 -> Switch/2, "Magnitude "/1

== matlab function RocketSimulation/Orbital Mechanics Calculations/MATLAB Function ==
  data: OrbitVelocity input; OrbitData output; Position input
function OrbitData = fcn(OrbitVelocity,Position)
